simulink model "FOC_SMO_PLL"  (R2022a)
settings: Solver=VariableStepDiscrete  StartTime=0.0  StopTime=1  RelTol=1e-5
InitFcn:
  | f=2000;
  | m=0.8;
  | Ts=1/f;
  | Vdc=48;
libraries: spsControlledVoltageSourceLib x3, simulink x3, slpidlib x2, spsDCVoltageSourceLib x1, spsPermanentMagnetSynchronousMachineLib x1, spsUniversalBridgeLib x1, spspowerguiLib x1
settings Model: Creator=XieXW  LastModifiedBy=XieXW

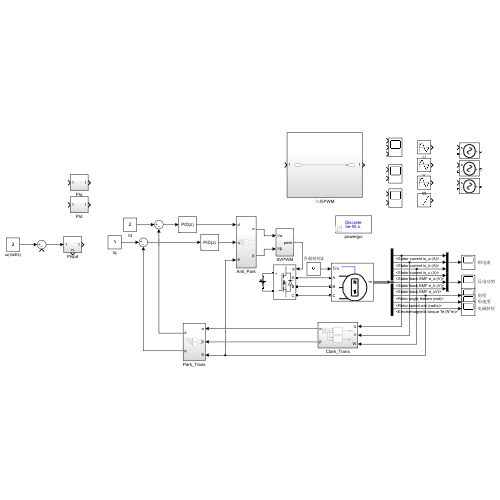
[thumbnail: Simulink's stored preview of the top-level diagram]
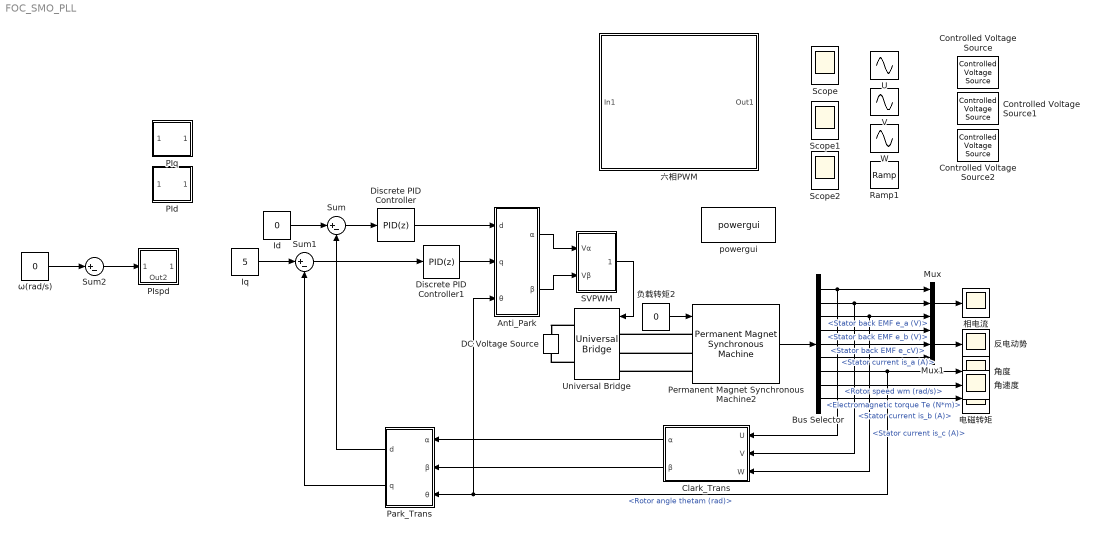
== system FOC_SMO_PLL ==
  Anti_Park : Subsystem
  Bus Selector : BusSelector  OutputSignals=Stator current is_a (A),Stator current is_b (A),Stator current is_c (A),Stator back EMF e_a (V),Stator back EMF e_b (V),Stator back EMF e_cV),Rotor angle thetam (rad),Rotor speed wm (rad/s),Electromagnetic torque Te (N*m)
  Clark_Trans : Subsystem
  Controlled Voltage Source : spsControlledVoltageSourceLib/Controlled Voltage Source  Initialize=on  Source_Type=AC  Amplitude=0  Phase=0  Frequency=0  Measurements=None
  Controlled Voltage Source1 : spsControlledVoltageSourceLib/Controlled Voltage Source  Initialize=on  Source_Type=AC  Amplitude=0  Phase=0  Frequency=0  Measurements=None
  Controlled Voltage Source2 : spsControlledVoltageSourceLib/Controlled Voltage Source  Initialize=on  Source_Type=AC  Amplitude=0  Phase=0  Frequency=0  Measurements=None
  DC Voltage Source : spsDCVoltageSourceLib/DC Voltage Source  Amplitude=Vdc  Measurements=None
  Discrete PID Controller : slpidlib/PID Controller  Controller=PID  Form=Parallel  TimeDomain=Discrete-time  UseExternalTs=off  SampleTime=-1  IntegratorMethod=Forward Euler  FilterMethod=Forward Euler  ControllerParametersSource=internal  P=0.5  I=500  UseKiTs=off  D=0  N=100  UseFilter=on  TunerSelectOption=Transfer Function Based (PID Tuner App)  InitialConditionSource=internal  InitialConditionForIntegrator=0  InitialConditionForFilter=0  DifferentiatorICPrevScaledInput=0  ExternalReset=none  TrackingMode=off  Kt=1  LimitOutput=off  SatLimitsSource=internal  UpperSaturationLimit=1  LowerSaturationLimit=-1  LinearizeAsGain=off  AntiWindupMode=none  Kb=1  POutMin=[]  POutMax=[]  IOutMin=[]  IOutMax=[]  DOutMin=[]  DOutMax=[]  NOutMin=[]  NOutMax=[]  SumOutMin=[]  SumOutMax=[]  SaturationOutMin=[]  SaturationOutMax=[]  PParamMin=[]  PParamMax=[]  IParamMin=[]  IParamMax=[]  DParamMin=[]  DParamMax=[]  NParamMin=[]  NParamMax=[]  KbParamMin=[]  KbParamMax=[]  KtParamMin=[]  KtParamMax=[]  KbOutMin=[]  KbOutMax=[]  KtOutMin=[]  KtOutMax=[]  IntegratorOutMin=[]  IntegratorOutMax=[]  FilterOutMin=[]  FilterOutMax=[]  SumI1OutMin=[]  SumI1OutMax=[]  SumI2OutMin=[]  SumI2OutMax=[]  SumI3OutMin=[]  SumI3OutMax=[]  SumI4OutMin=[]  SumI4OutMax=[]  SumDOutMin=[]  SumDOutMax=[]  DifferentiatorOutMin=[]  DifferentiatorOutMax=[]  FilterDiffOutCoefMin=[]  FilterDiffOutCoefMax=[]  ReciprocalOutMin=[]  ReciprocalOutMax=[]  SumDenOutMin=[]  SumDenOutMax=[]  SumNumOutMin=[]  SumNumOutMax=[]  DivideOutMin=[]  DivideOutMax=[]  UdiffTsProdOutMin=[]  UdiffTsProdOutMax=[]  NTsProdOutMin=[]  NTsProdOutMax=[]  UintegralTsProdOutMin=[]  UintegralTsProdOutMax=[]  UngainTsProdOutMin=[]  UngainTsProdOutMax=[]  IntegratorContinuousStateAttributes=''  IntegratorStateMustResolveToSignalObject=off  IntegratorRTWStateStorageClass=Auto  FilterContinuousStateAttributes=''  FilterStateMustResolveToSignalObject=off  FilterRTWStateStorageClass=Auto  ParallelPVariant=InternalParameters  IdealPVariant=Disabled  IVariant=InternalParameters  DVariant=InternalParameters  IntegratorVariant=Discrete  SatVariant=Disabled  AWVariant=Passthrough  PCopyVariant=Disabled  TRVariant=Disabled  FdbkBlocksVariant=Forward  IdealPFdbkVariant=Disabled  SatFdbkVariant=Disabled  DerivativeFilterVariant=ForwardEulerFilter  NVariant=InternalParameters  NCopyVariant=Disabled  FilterICVariant=InternalICsFilter  IntegratorICVariant=InternalICs  ExternalResetVariant=Disabled  TRSumVariant=Passthrough  SumFdbkVariant=Disabled  SumVariant=Sum_PID  TsampFilterVariant=InternalTs  TsampNgainVariant=Passthrough  TsampIntegralVariant=Passthrough  ExternalSaturationOutDataTypeStr=Inherit: Same as second input  aMode=0
  Discrete PID Controller1 : slpidlib/PID Controller  Controller=PID  Form=Parallel  TimeDomain=Discrete-time  UseExternalTs=off  SampleTime=-1  IntegratorMethod=Forward Euler  FilterMethod=Forward Euler  ControllerParametersSource=internal  P=0.5  I=500  UseKiTs=off  D=0  N=100  UseFilter=on  TunerSelectOption=Transfer Function Based (PID Tuner App)  InitialConditionSource=internal  InitialConditionForIntegrator=0  InitialConditionForFilter=0  DifferentiatorICPrevScaledInput=0  ExternalReset=none  TrackingMode=off  Kt=1  LimitOutput=off  SatLimitsSource=internal  UpperSaturationLimit=1  LowerSaturationLimit=-1  LinearizeAsGain=off  AntiWindupMode=none  Kb=1  POutMin=[]  POutMax=[]  IOutMin=[]  IOutMax=[]  DOutMin=[]  DOutMax=[]  NOutMin=[]  NOutMax=[]  SumOutMin=[]  SumOutMax=[]  SaturationOutMin=[]  SaturationOutMax=[]  PParamMin=[]  PParamMax=[]  IParamMin=[]  IParamMax=[]  DParamMin=[]  DParamMax=[]  NParamMin=[]  NParamMax=[]  KbParamMin=[]  KbParamMax=[]  KtParamMin=[]  KtParamMax=[]  KbOutMin=[]  KbOutMax=[]  KtOutMin=[]  KtOutMax=[]  IntegratorOutMin=[]  IntegratorOutMax=[]  FilterOutMin=[]  FilterOutMax=[]  SumI1OutMin=[]  SumI1OutMax=[]  SumI2OutMin=[]  SumI2OutMax=[]  SumI3OutMin=[]  SumI3OutMax=[]  SumI4OutMin=[]  SumI4OutMax=[]  SumDOutMin=[]  SumDOutMax=[]  DifferentiatorOutMin=[]  DifferentiatorOutMax=[]  FilterDiffOutCoefMin=[]  FilterDiffOutCoefMax=[]  ReciprocalOutMin=[]  ReciprocalOutMax=[]  SumDenOutMin=[]  SumDenOutMax=[]  SumNumOutMin=[]  SumNumOutMax=[]  DivideOutMin=[]  DivideOutMax=[]  UdiffTsProdOutMin=[]  UdiffTsProdOutMax=[]  NTsProdOutMin=[]  NTsProdOutMax=[]  UintegralTsProdOutMin=[]  UintegralTsProdOutMax=[]  UngainTsProdOutMin=[]  UngainTsProdOutMax=[]  IntegratorContinuousStateAttributes=''  IntegratorStateMustResolveToSignalObject=off  IntegratorRTWStateStorageClass=Auto  FilterContinuousStateAttributes=''  FilterStateMustResolveToSignalObject=off  FilterRTWStateStorageClass=Auto  ParallelPVariant=InternalParameters  IdealPVariant=Disabled  IVariant=InternalParameters  DVariant=InternalParameters  IntegratorVariant=Discrete  SatVariant=Disabled  AWVariant=Passthrough  PCopyVariant=Disabled  TRVariant=Disabled  FdbkBlocksVariant=Forward  IdealPFdbkVariant=Disabled  SatFdbkVariant=Disabled  DerivativeFilterVariant=ForwardEulerFilter  NVariant=InternalParameters  NCopyVariant=Disabled  FilterICVariant=InternalICsFilter  IntegratorICVariant=InternalICs  ExternalResetVariant=Disabled  TRSumVariant=Passthrough  SumFdbkVariant=Disabled  SumVariant=Sum_PID  TsampFilterVariant=InternalTs  TsampNgainVariant=Passthrough  TsampIntegralVariant=Passthrough  ExternalSaturationOutDataTypeStr=Inherit: Same as second input  aMode=0
  Id : Constant  Value=0
  Iq : Constant  Value=5
  Mux : Mux  Inputs=3
  Mux1 : Mux  Inputs=3
  PId : Subsystem
  PIq : Subsystem
  PIspd : Subsystem
      settings: PortSchema="{\"entries\":[{\"content\":{\"sides\":[{\"content\":{\"connectorIds\":[\"In1\"]},\"type\":\"ConnectorPlacement.EquallySpacedRectSide\",\"uuid\":\"86a8a1bc-41cc-400f-8a05-3a947add3d03\"},{\"content\":{\"connectorIds\":[\"Out1\"],\"side\":\"RIGHT\"},\"type\":\"ConnectorPlacement.EquallySpacedRectSide\",\"uuid\":\"9c1cbacf-2414-4d8a-8256-d876bc22501c\"},{\"content\":{\"connectorIds\":[],\"side\":\"TOP\"},\"type\":\"ConnectorPlacement.EquallySpacedRectSide\",\"uuid\":\"6e387cc1-f2da-4b1b-b101-a7ee69ec67bc\"},{\"content\":{\"connectorIds\":[\"Out2\"],\"side\":\"BOTTOM\"},\"type\":\"ConnectorPlacement.EquallySpacedRectSide\",\"uuid\":\"142bb7ea-360a-4ae3-b1bc-2d54ba528d2c\"}]},\"type\":\"ConnectorPlacement.EquallySpacedConnector\",\"uuid\":\"a78a607e-a50e-44f4-91e4-2b5711de5b78\"}],\"packageUris\":[\"http://schema.mathworks.com/mf0/Connector/R2020b\"],\"version\":\"1.0\"}"
  Park_Trans : Subsystem
  Permanent Magnet Synchronous Machine2 : spsPermanentMagnetSynchronousMachineLib/Permanent Magnet Synchronous Machine  NbPhases=3  FluxDistribution=Trapezoidal  RotorType=Round  MechanicalLoad=Torque Tm  PresetModel=No  ShowDetailedParameters=on  MeasurementBus=off  Resistance=0.0485  Inductance=8.5e-3  dqInductances=[8.5e-3,8.5e-3]  La=0.000395  MachineConstant=Flux linkage established by magnets (V.s)  Flux=0.1194  VoltageCst=25.0071  TorqueCst=0.2388  Flat=120  Mechanical=[0.0027 0.0124924 1 0]  PolePairs=4  InitialConditions=[0,0, 0,0]  InitialConditions5ph=[0 0 0 0 0 0]  RefAngle=Aligned with phase A axis (original Park)  IterativeDiscreteModel=Trapezoidal non iterative  TsBlock=-1  TsPowergui=0
  Ramp1 : simulink/Sources/Ramp  slope=-pi/2  start=0  InitialOutput=0
  SVPWM : Subsystem
  Scope : Scope  NumInputPorts=3
  Scope1 : Scope  NumInputPorts=2
  Scope2 : Scope  NumInputPorts=2
  Sum : Sum  Inputs=|+-
  Sum1 : Sum  Inputs=|+-
  Sum2 : Sum  Inputs=|+-
  U : Sin  Frequency=pi/2  SampleTime=0
  Universal Bridge : spsUniversalBridgeLib/Universal Bridge  Arms=3  SnubberResistance=1e5  SnubberCapacitance=inf  Device=MOSFET / Diodes  Ron=1e-3  Lon=0  ForwardVoltages="[  0  0  ]"  ForwardVoltage=0  GTOparameters=[ 10e-6 , 20e-6 ]  IGBTparameters=[ 1e-6 , 2e-6 ]  Measurements=None  Measurements_2=None  converterType=Rectifier
  V : Sin  Frequency=pi/2  Phase=2*pi/3  SampleTime=0
  W : Sin  Frequency=pi/2  Phase=-2*pi/3  SampleTime=0
  powergui : spspowerguiLib/powergui  Priority=1  SimulationMode=Discrete  SampleTime=50e-6  frequency=60  Iterations=50  frequencyindice=0  Pbase=100e6  ErrMax=1e-4  UnitsV=kV  UnitsW=MW  buscounter=0  FunctionMessages=off  echomessages=off  EnableUseOfTLC=off  CurrentSourceSwitches=off  DisableSnubberDevices=off  DisableRonSwitches=off  DisableVfSwitches=off  DisplayEquations=off  AutomaticDiscreteSolvers=off  SolverType=Tustin/Backward Euler (TBE)  Interpol=off  ExternalGateDelay=off  methode=off  Ts=100  x0status=blocks  SPID=on  SwTol=0  HookPort=off  NonlinearTolerance=1e-4  nMaxIteration=100  ContinueOnMaxIteration=off  RestoreLinks=warning  ResistiveCurrentMeasurement=off  Frange=[0:2:500]  Ylog=off  Xlog=on  ShowGrid=off  save=off  variable=ZData  structure=0  ZoomFFT=off  StartTime=0.0  cycles=1  DisplayStyle=1  fundamental=60  FreqAxis=off  MaxFrequency=1000  frequencyindicesteady=1  RmsSteady=1  display=off
  ω(rad/s) : Constant  Value=0
  六相PWM : Subsystem
  反电动势 : Scope
  电磁转矩 : Scope
  相电流 : Scope
  角度 : Scope
  角速度 : Scope
  负载转矩2 : Constant  Value=0
  wires:
  Anti_Park/1(α) -> SVPWM/1(Vα)
  Anti_Park/2(β) -> SVPWM/2(Vβ)
  Clark_Trans/1(α) -> Park_Trans/1(α)
  Clark_Trans/2(β) -> Park_Trans/2(β)
  Id/1 -> Sum/1
  Park_Trans/1(d) -> Sum/2
  Park_Trans/2(q) -> Sum1/2
  Sum2/1 -> PIspd/1(In1)
  ω(rad/s)/1 -> Sum2/1
  Iq/1 -> Sum1/1
  Discrete PID Controller/1 -> Anti_Park/1(d)
  Sum/1 -> Discrete PID Controller/1
  Discrete PID Controller1/1 -> Anti_Park/2(q)
  Sum1/1 -> Discrete PID Controller1/1
  Bus Selector/2 -> Clark_Trans/2(V), Mux/2  "<Stator current is_b (A)>"
  Bus Selector/1 -> Clark_Trans/1(U), Mux/1  "<Stator current is_a (A)>"
  Bus Selector/3 -> Clark_Trans/3(W), Mux/3  "<Stator current is_c (A)>"
  Mux/1 -> 相电流/1
  Bus Selector/4 -> Mux1/1  "<Stator back EMF e_a (V)>"
  Bus Selector/5 -> Mux1/2  "<Stator back EMF e_b (V)>"
  Bus Selector/6 -> Mux1/3  "<Stator back EMF e_cV)>"
  Mux1/1 -> 反电动势/1
  Bus Selector/9 -> 电磁转矩/1  "<Electromagnetic torque Te (N*m)>"
  Bus Selector/7 -> 角度/1, Park_Trans/3(θ), Anti_Park/3(θ)  "<Rotor angle thetam (rad)>"
  Bus Selector/8 -> 角速度/1  "<Rotor speed wm (rad/s)>"
  SVPWM/1(pwm) -> Universal Bridge/1
  负载转矩2/1 -> Permanent Magnet Synchronous Machine2/1
  Permanent Magnet Synchronous Machine2/1 -> Bus Selector/1
  connections:
  Universal Bridge/RConn1 -- DC Voltage Source/RConn1
  Universal Bridge/RConn2 -- DC Voltage Source/LConn1
  Permanent Magnet Synchronous Machine2/LConn1 -- Universal Bridge/LConn1
  Permanent Magnet Synchronous Machine2/LConn2 -- Universal Bridge/LConn2
  Permanent Magnet Synchronous Machine2/LConn3 -- Universal Bridge/LConn3

== system FOC_SMO_PLL/Anti_Park ==
  d : Inport
  q : Inport  Port=2
  θ : Inport  Port=3
  MATLAB Function1 : MATLAB Function  TreatAsAtomicUnit=on
  MATLAB Function2 : MATLAB Function  TreatAsAtomicUnit=on
  α : Outport
  β : Outport  Port=2
  wires:
  MATLAB Function1/1(alpha) -> α/1
  d/1 -> MATLAB Function2/1(d), MATLAB Function1/1(d)
  q/1 -> MATLAB Function2/2(q), MATLAB Function1/2(q)
  θ/1 -> MATLAB Function2/3(angle), MATLAB Function1/3(angle)
  MATLAB Function2/1(beta) -> β/1

== system FOC_SMO_PLL/Clark_Trans ==
  U : Inport
  V : Inport  Port=2
  W : Inport  Port=3
  MATLAB Function : MATLAB Function  TreatAsAtomicUnit=on
  MATLAB Function1 : MATLAB Function  TreatAsAtomicUnit=on
  α : Outport
  β : Outport  Port=2
  wires:
  U/1 -> MATLAB Function/1(u)
  V/1 -> MATLAB Function1/1(v), MATLAB Function/2(v)
  W/1 -> MATLAB Function1/2(w), MATLAB Function/3(w)
  MATLAB Function/1(alpha) -> α/1
  MATLAB Function1/1(beta) -> β/1

== system FOC_SMO_PLL/PId ==
  In1 : Inport
  Out1 : Outport
  wires:
  In1/1 -> Out1/1

== system FOC_SMO_PLL/PIq ==
  In1 : Inport
  Out1 : Outport
  wires:
  In1/1 -> Out1/1

== system FOC_SMO_PLL/PIspd ==
  In1 : Inport
  Out1 : Outport
  Out2 : Outport  Port=2
  wires:
  In1/1 -> Out1/1

== system FOC_SMO_PLL/Park_Trans ==
  α : Inport
  β : Inport  Port=2
  θ : Inport  Port=3
  MATLAB Function : MATLAB Function  TreatAsAtomicUnit=on
  MATLAB Function1 : MATLAB Function  TreatAsAtomicUnit=on
  d : Outport
  q : Outport  Port=2
  wires:
  α/1 -> MATLAB Function/1(alpha), MATLAB Function1/1(alpha)
  MATLAB Function1/1(d) -> d/1
  β/1 -> MATLAB Function/2(beta), MATLAB Function1/2(beta)
  MATLAB Function/1(q) -> q/1
  θ/1 -> MATLAB Function/3(angle), MATLAB Function1/3(angle)

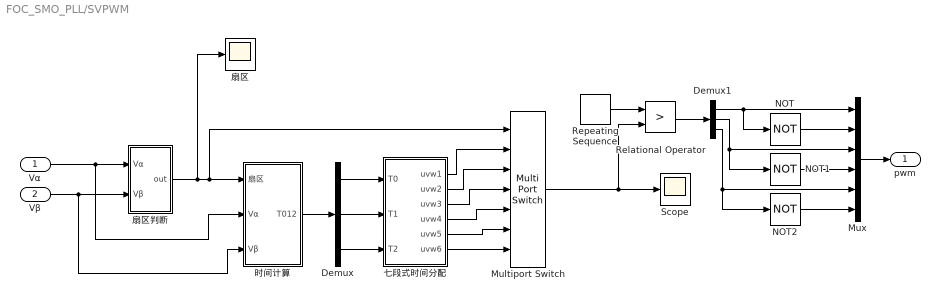
== system FOC_SMO_PLL/SVPWM ==
  Vα : Inport
  Vβ : Inport  Port=2
  Demux : Demux  Outputs=3
  Demux1 : Demux  Outputs=3
  Multiport Switch : MultiPortSwitch  Inputs=6  SaturateOnIntegerOverflow=off  InputSameDT=off
  Mux : Mux  Inputs=6
  NOT : Logic  Operator=NOT  IconShape=distinctive  AllPortsSameDT=off  OutDataTypeStr=boolean
  NOT1 : Logic  Operator=NOT  IconShape=distinctive  AllPortsSameDT=off  OutDataTypeStr=boolean
  NOT2 : Logic  Operator=NOT  IconShape=distinctive  AllPortsSameDT=off  OutDataTypeStr=boolean
  Relational Operator : RelationalOperator  Operator=>  OutDataTypeStr=boolean  RndMeth=Simplest  InputSameDT=off
  Repeating Sequence : simulink/Sources/Repeating Sequence  rep_seq_t=[0 Ts/2 Ts]  rep_seq_y=[0 1 0]
  Scope : Scope
  七段式时间分配 : Subsystem
  扇区 : Scope
  扇区判断 : Subsystem
  时间计算 : Subsystem
  pwm : Outport
  wires:
  七段式时间分配/6(uvw6) -> Multiport Switch/7
  Demux1/3 -> NOT2/1, Mux/5
  七段式时间分配/5(uvw5) -> Multiport Switch/6
  Demux1/2 -> NOT1/1, Mux/3
  Relational Operator/1 -> Demux1/1
  Demux/1 -> 七段式时间分配/1(T0)
  扇区判断/1(out) -> Multiport Switch/1, 时间计算/1(扇区), 扇区/1
  七段式时间分配/2(uvw2) -> Multiport Switch/3
  Vα/1 -> 时间计算/2(Vα), 扇区判断/1(Vα)
  Vβ/1 -> 时间计算/3(Vβ), 扇区判断/2(Vβ)
  七段式时间分配/1(uvw1) -> Multiport Switch/2
  时间计算/1(T012) -> Demux/1
  七段式时间分配/4(uvw4) -> Multiport Switch/5
  Demux/2 -> 七段式时间分配/2(T1)
  Multiport Switch/1 -> Relational Operator/2, Scope/1
  七段式时间分配/3(uvw3) -> Multiport Switch/4
  Demux/3 -> 七段式时间分配/3(T2)
  Repeating Sequence/1 -> Relational Operator/1
  Demux1/1 -> Mux/1, NOT/1
  NOT2/1 -> Mux/6
  NOT1/1 -> Mux/4
  NOT/1 -> Mux/2
  Mux/1 -> pwm/1

== system FOC_SMO_PLL/六相PWM ==
  In1 : Inport
  Out1 : Outport
  wires:
  In1/1 -> Out1/1

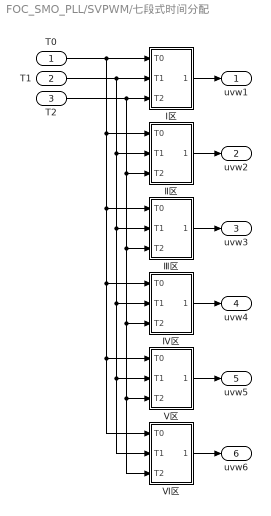
== system FOC_SMO_PLL/SVPWM/七段式时间分配 ==
  T0 : Inport
  T1 : Inport  Port=2
  T2 : Inport  Port=3
  Ⅰ区 : Subsystem
  Ⅱ区 : Subsystem
  Ⅲ区 : Subsystem
  Ⅳ区 : Subsystem
  Ⅴ区 : Subsystem
  Ⅵ区 : Subsystem
  uvw1 : Outport
  uvw2 : Outport  Port=2
  uvw3 : Outport  Port=3
  uvw4 : Outport  Port=4
  uvw5 : Outport  Port=5
  uvw6 : Outport  Port=6
  wires:
  Ⅱ区/1(uvw2) -> uvw2/1
  T1/1 -> Ⅵ区/2(T1), Ⅴ区/2(T1), Ⅳ区/2(T1), Ⅲ区/2(T1), Ⅱ区/2(T1), Ⅰ区/2(T1)
  Ⅰ区/1(uvw1) -> uvw1/1
  T2/1 -> Ⅵ区/3(T2), Ⅴ区/3(T2), Ⅳ区/3(T2), Ⅲ区/3(T2), Ⅱ区/3(T2), Ⅰ区/3(T2)
  Ⅳ区/1(uvw4) -> uvw4/1
  T0/1 -> Ⅱ区/1(T0), Ⅵ区/1(T0), Ⅴ区/1(T0), Ⅳ区/1(T0), Ⅲ区/1(T0), Ⅰ区/1(T0)
  Ⅵ区/1(uvw6) -> uvw6/1
  Ⅲ区/1(uvw3) -> uvw3/1
  Ⅴ区/1(uvw5) -> uvw5/1

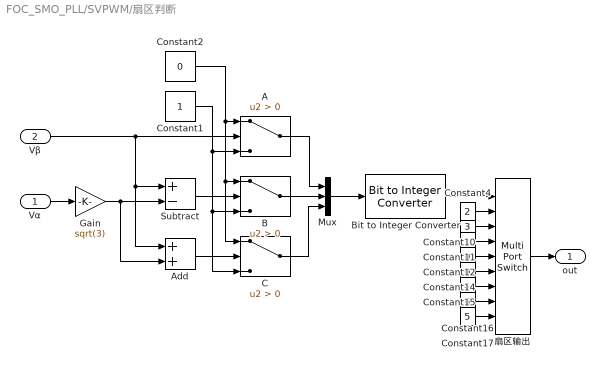
== system FOC_SMO_PLL/SVPWM/扇区判断 ==
  Vα : Inport
  Vβ : Inport  Port=2
  A : Switch  Criteria=u2 > Threshold  SaturateOnIntegerOverflow=off  InputSameDT=off
  Add : Sum
  B : Switch  Criteria=u2 > Threshold  SaturateOnIntegerOverflow=off  InputSameDT=off
  Bit to Integer Converter : simulink/Logic and Bit Operations/Bit to Integer Converter  nbits=3  bitOrder=MSB first  signedOutputValues=Unsigned  outDtype=Inherit via internal rule  outDtypeSigned=Inherit via internal rule
      settings: SourceProductBaseCode=SL
  C : Switch  Criteria=u2 > Threshold  SaturateOnIntegerOverflow=off  InputSameDT=off
  Constant1 : Constant
  Constant10 : Constant  Value=3
  Constant11 : Constant
  Constant12 : Constant  Value=0
  Constant14 : Constant  Value=0
  Constant15 : Constant  Value=4
  Constant16 : Constant  Value=6
  Constant17 : Constant  Value=5
  Constant2 : Constant  Value=0
  Constant4 : Constant  Value=2
  Gain : Gain  Gain=sqrt(3)
  Mux : Mux  Inputs=3
  Subtract : Sum  Inputs=+-
  扇区输出 : MultiPortSwitch  DataPortOrder=Zero-based contiguous  Inputs=8  zeroidx=on  SaturateOnIntegerOverflow=off  InputSameDT=off
  out : Outport
  wires:
  A/1 -> Mux/1
  Vβ/1 -> A/2, Add/1, Subtract/1
  Mux/1 -> Bit to Integer Converter/1
  Subtract/1 -> B/2
  B/1 -> Mux/2
  Constant2/1 -> C/1, B/1, A/1
  Gain/1 -> Add/2, Subtract/2
  Constant1/1 -> C/3, B/3, A/3
  C/1 -> Mux/3
  Add/1 -> C/2
  Vα/1 -> Gain/1
  扇区输出/1 -> out/1
  Bit to Integer Converter/1 -> 扇区输出/1
  Constant4/1 -> 扇区输出/2
  Constant10/1 -> 扇区输出/3
  Constant11/1 -> 扇区输出/4
  Constant12/1 -> 扇区输出/5
  Constant14/1 -> 扇区输出/6
  Constant15/1 -> 扇区输出/7
  Constant16/1 -> 扇区输出/8
  Constant17/1 -> 扇区输出/9

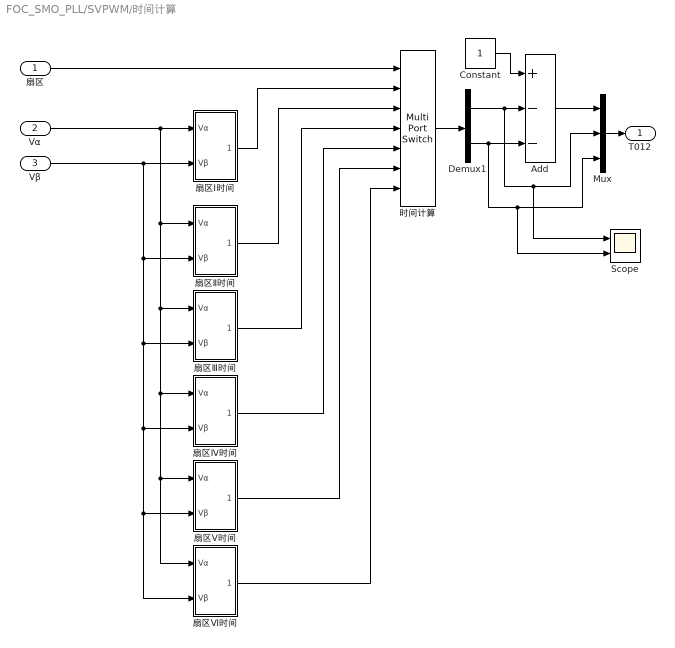
== system FOC_SMO_PLL/SVPWM/时间计算 ==
  扇区 : Inport
  Vα : Inport  Port=2
  Vβ : Inport  Port=3
  Add : Sum  Inputs=+--
  Constant : Constant
  Demux1 : Demux  Outputs=2
  Mux : Mux  Inputs=3
  Scope : Scope  NumInputPorts=2
  扇区Ⅰ时间 : Subsystem
  扇区Ⅱ时间 : Subsystem
  扇区Ⅲ时间 : Subsystem
  扇区Ⅳ时间 : Subsystem
  扇区Ⅴ时间 : Subsystem
  扇区Ⅵ时间 : Subsystem
  时间计算 : MultiPortSwitch  Inputs=6  SaturateOnIntegerOverflow=off  InputSameDT=off
  T012 : Outport
  wires:
  Vα/1 -> 扇区Ⅵ时间/1(Vα), 扇区Ⅴ时间/1(Vα), 扇区Ⅳ时间/1(Vα), 扇区Ⅲ时间/1(Vα), 扇区Ⅱ时间/1(Vα), 扇区Ⅰ时间/1(Vα)
  时间计算/1 -> Demux1/1
  Demux1/1 -> Scope/1, Mux/2, Add/2
  Add/1 -> Mux/1
  Demux1/2 -> Scope/2, Mux/3, Add/3
  Vβ/1 -> 扇区Ⅵ时间/2(Vβ), 扇区Ⅴ时间/2(Vβ), 扇区Ⅳ时间/2(Vβ), 扇区Ⅲ时间/2(Vβ), 扇区Ⅱ时间/2(Vβ), 扇区Ⅰ时间/2(Vβ)
  Constant/1 -> Add/1
  扇区Ⅰ时间/1(Tout1) -> 时间计算/2
  扇区Ⅴ时间/1(Tout5) -> 时间计算/6
  扇区Ⅳ时间/1(Tout4) -> 时间计算/5
  扇区Ⅱ时间/1(Tout2) -> 时间计算/3
  Mux/1 -> T012/1
  扇区Ⅵ时间/1(Tout6) -> 时间计算/7
  扇区Ⅲ时间/1(Tout3) -> 时间计算/4
  扇区/1 -> 时间计算/1

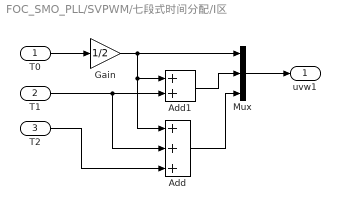
== system FOC_SMO_PLL/SVPWM/七段式时间分配/Ⅰ区 ==
  T0 : Inport
  T1 : Inport  Port=2
  T2 : Inport  Port=3
  Add : Sum  Inputs=+++
  Add1 : Sum
  Gain : Gain  Gain=1/2
  Mux : Mux  Inputs=3
  uvw1 : Outport
  wires:
  Add/1 -> Mux/3
  Gain/1 -> Add/1, Add1/1, Mux/1
  Add1/1 -> Mux/2
  T1/1 -> Add/2, Add1/2
  Mux/1 -> uvw1/1
  T2/1 -> Add/3
  T0/1 -> Gain/1

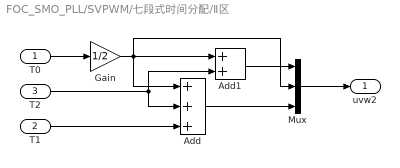
== system FOC_SMO_PLL/SVPWM/七段式时间分配/Ⅱ区 ==
  T0 : Inport
  T1 : Inport  Port=2
  T2 : Inport  Port=3
  Add : Sum  Inputs=+++
  Add1 : Sum
  Gain : Gain  Gain=1/2
  Mux : Mux  Inputs=3
  uvw2 : Outport
  wires:
  Mux/1 -> uvw2/1
  T0/1 -> Gain/1
  Gain/1 -> Add/1, Mux/2, Add1/1
  T2/1 -> Add/2, Add1/2
  Add1/1 -> Mux/1
  T1/1 -> Add/3
  Add/1 -> Mux/3

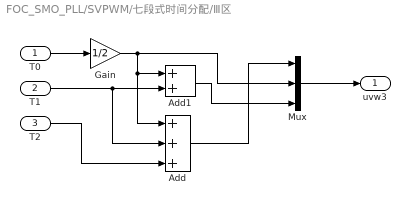
== system FOC_SMO_PLL/SVPWM/七段式时间分配/Ⅲ区 ==
  T0 : Inport
  T1 : Inport  Port=2
  T2 : Inport  Port=3
  Add : Sum  Inputs=+++
  Add1 : Sum
  Gain : Gain  Gain=1/2
  Mux : Mux  Inputs=3
  uvw3 : Outport
  wires:
  T0/1 -> Gain/1
  T2/1 -> Add/3
  Mux/1 -> uvw3/1
  T1/1 -> Add1/2, Add/2
  Gain/1 -> Mux/2, Add1/1, Add/1
  Add/1 -> Mux/1
  Add1/1 -> Mux/3

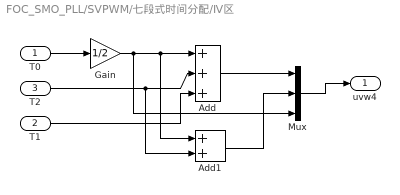
== system FOC_SMO_PLL/SVPWM/七段式时间分配/Ⅳ区 ==
  T0 : Inport
  T1 : Inport  Port=2
  T2 : Inport  Port=3
  Add : Sum  Inputs=+++
  Add1 : Sum
  Gain : Gain  Gain=1/2
  Mux : Mux  Inputs=3
  uvw4 : Outport
  wires:
  Gain/1 -> Add/1, Add1/1, Mux/3
  T0/1 -> Gain/1
  Mux/1 -> uvw4/1
  T2/1 -> Add1/2, Add/2
  T1/1 -> Add/3
  Add/1 -> Mux/1
  Add1/1 -> Mux/2

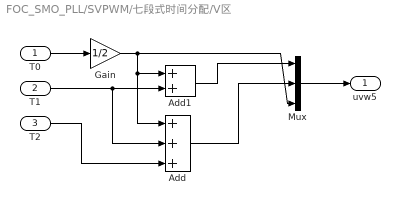
== system FOC_SMO_PLL/SVPWM/七段式时间分配/Ⅴ区 ==
  T0 : Inport
  T1 : Inport  Port=2
  T2 : Inport  Port=3
  Add : Sum  Inputs=+++
  Add1 : Sum
  Gain : Gain  Gain=1/2
  Mux : Mux  Inputs=3
  uvw5 : Outport
  wires:
  Gain/1 -> Add/1, Add1/1, Mux/3
  T1/1 -> Add/2, Add1/2
  Mux/1 -> uvw5/1
  T2/1 -> Add/3
  T0/1 -> Gain/1
  Add/1 -> Mux/2
  Add1/1 -> Mux/1

== system FOC_SMO_PLL/SVPWM/七段式时间分配/Ⅵ区 ==
  T0 : Inport
  T1 : Inport  Port=2
  T2 : Inport  Port=3
  Add : Sum  Inputs=+++
  Add1 : Sum
  Gain : Gain  Gain=1/2
  Mux : Mux  Inputs=3
  uvw6 : Outport
  wires:
  Mux/1 -> uvw6/1
  T0/1 -> Gain/1
  Gain/1 -> Add/1, Add1/2, Mux/1
  T2/1 -> Add/2, Add1/1
  T1/1 -> Add/3
  Add/1 -> Mux/2
  Add1/1 -> Mux/3

== system FOC_SMO_PLL/SVPWM/时间计算/扇区Ⅰ时间 ==
  Vα : Inport
  Vβ : Inport  Port=2
  Gain : Gain  Gain=1/2
  Mux : Mux  Inputs=2
  Subtract : Sum  Inputs=+-
  sqrt(3)/2 : Gain  Gain=sqrt(3)/2
  Tout1 : Outport
  wires:
  Gain/1 -> Subtract/2
  Vβ/1 -> Mux/2, Gain/1
  Subtract/1 -> Mux/1
  Mux/1 -> Tout1/1
  sqrt(3)/2/1 -> Subtract/1
  Vα/1 -> sqrt(3)/2/1

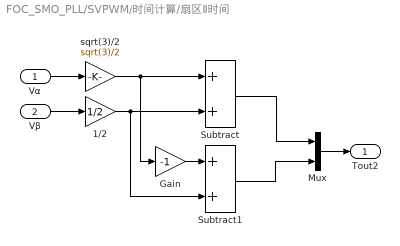
== system FOC_SMO_PLL/SVPWM/时间计算/扇区Ⅱ时间 ==
  Vα : Inport
  Vβ : Inport  Port=2
  1/2 : Gain  Gain=1/2
  Gain : Gain  Gain=-1
  Mux : Mux  Inputs=2
  Subtract : Sum
  Subtract1 : Sum
  sqrt(3)/2 : Gain  Gain=sqrt(3)/2
  Tout2 : Outport
  wires:
  Vα/1 -> sqrt(3)/2/1
  Mux/1 -> Tout2/1
  Subtract/1 -> Mux/1
  Vβ/1 -> 1/2/1
  1/2/1 -> Subtract1/2, Subtract/2
  sqrt(3)/2/1 -> Gain/1, Subtract/1
  Subtract1/1 -> Mux/2
  Gain/1 -> Subtract1/1

== system FOC_SMO_PLL/SVPWM/时间计算/扇区Ⅲ时间 ==
  Vα : Inport
  Vβ : Inport  Port=2
  1/2 : Gain  Gain=1/2
  Gain : Gain  Gain=-1
  Mux : Mux  Inputs=2
  Subtract1 : Sum
  sqrt(3)/2 : Gain  Gain=sqrt(3)/2
  Tout3 : Outport
  wires:
  Vβ/1 -> Mux/1, 1/2/1
  Mux/1 -> Tout3/1
  Vα/1 -> sqrt(3)/2/1
  sqrt(3)/2/1 -> Subtract1/1
  1/2/1 -> Subtract1/2
  Subtract1/1 -> Gain/1
  Gain/1 -> Mux/2

== system FOC_SMO_PLL/SVPWM/时间计算/扇区Ⅳ时间 ==
  Vα : Inport
  Vβ : Inport  Port=2
  -sqrt(3)/2 : Gain  Gain=-sqrt(3)/2
  1/2 : Gain  Gain=1/2
  Gain : Gain  Gain=-1
  Mux : Mux  Inputs=2
  Subtract : Sum
  Tout4 : Outport
  wires:
  Vα/1 -> -sqrt(3)/2/1
  Mux/1 -> Tout4/1
  Vβ/1 -> Gain/1, 1/2/1
  Gain/1 -> Mux/2
  1/2/1 -> Subtract/2
  -sqrt(3)/2/1 -> Subtract/1
  Subtract/1 -> Mux/1

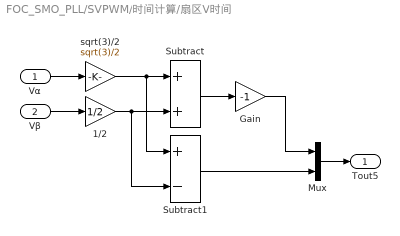
== system FOC_SMO_PLL/SVPWM/时间计算/扇区Ⅴ时间 ==
  Vα : Inport
  Vβ : Inport  Port=2
  1/2 : Gain  Gain=1/2
  Gain : Gain  Gain=-1
  Mux : Mux  Inputs=2
  Subtract : Sum
  Subtract1 : Sum  Inputs=+-
  sqrt(3)/2 : Gain  Gain=sqrt(3)/2
  Tout5 : Outport
  wires:
  1/2/1 -> Subtract1/2, Subtract/2
  Vβ/1 -> 1/2/1
  Mux/1 -> Tout5/1
  Vα/1 -> sqrt(3)/2/1
  sqrt(3)/2/1 -> Subtract1/1, Subtract/1
  Subtract/1 -> Gain/1
  Gain/1 -> Mux/1
  Subtract1/1 -> Mux/2

== system FOC_SMO_PLL/SVPWM/时间计算/扇区Ⅵ时间 ==
  Vα : Inport
  Vβ : Inport  Port=2
  1/2 : Gain  Gain=1/2
  Gain : Gain  Gain=-1
  Mux : Mux  Inputs=2
  Subtract1 : Sum
  sqrt(3)/2 : Gain  Gain=sqrt(3)/2
  Tout6 : Outport
  wires:
  Vα/1 -> sqrt(3)/2/1
  sqrt(3)/2/1 -> Subtract1/1
  Mux/1 -> Tout6/1
  Vβ/1 -> Gain/1, 1/2/1
  1/2/1 -> Subtract1/2
  Subtract1/1 -> Mux/2
  Gain/1 -> Mux/1

== matlab function FOC_SMO_PLL/Clark_Trans/MATLAB Function ==
  data: u input; alpha output; v input; w input
function alpha = fcn(u,v,w)

alpha = (2/3)*(u+(-1/2)*v+(-1/2)*w);

== matlab function FOC_SMO_PLL/Park_Trans/MATLAB Function ==
  data: alpha input; q output; beta input; angle input
function q = fcn(alpha,beta,angle)

q = -alpha*sin(angle)+beta*cos(angle);

== matlab function FOC_SMO_PLL/Park_Trans/MATLAB Function1 ==
  data: alpha input; d output; beta input; angle input
function d = fcn(alpha,beta,angle)

d = alpha*cos(angle)+beta*sin(angle);

== matlab function FOC_SMO_PLL/Anti_Park/MATLAB Function1 ==
  data: d input; alpha output; q input; angle input
function alpha = fcn(d,q,angle)

alpha = d*cos(angle)-q*sin(angle);

== matlab function FOC_SMO_PLL/Anti_Park/MATLAB Function2 ==
  data: d input; beta output; q input; angle input
function beta = fcn(d,q,angle)

beta = d*sin(angle)+q*cos(angle);

== matlab function FOC_SMO_PLL/Clark_Trans/MATLAB Function1 ==
  data: beta output; v input; w input
function beta = fcn(v,w)

beta = (2/3)*((sqrt(3)/2)*v+(-sqrt(3)/2)*w);
